simulink library "BibSpielo"  (R2025b)
settings: Solver=VariableStepAuto  StartTime=0.0  StopTime=10.0  RelTol=1e-3
settings Model: Creator=henni  LastModifiedBy=henni

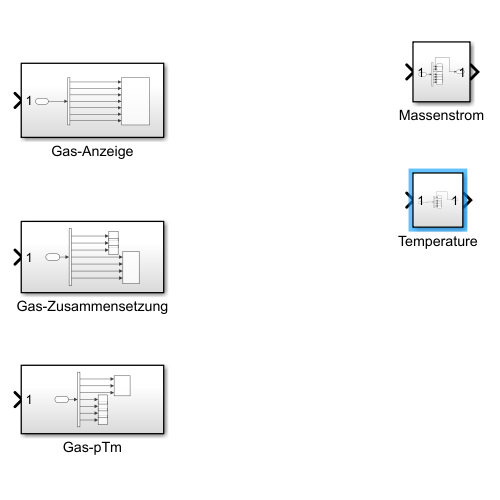
[thumbnail: Simulink's stored preview of the top-level diagram]
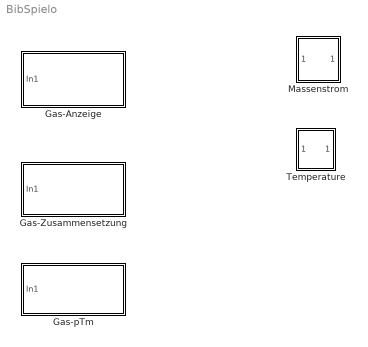
== system BibSpielo ==
  Gas-Anzeige : Subsystem
  Gas-Zusammensetzung : Subsystem
  Gas-pTm : Subsystem
  Massenstrom : Subsystem
  Temperature : Subsystem

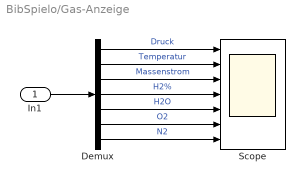
== system BibSpielo/Gas-Anzeige ==
  In1 : Inport
  Demux : Demux  Outputs=7
  Scope : Scope  NumInputPorts=7
  wires:
  Demux/3 -> Scope/3  "Massenstrom"
  Demux/2 -> Scope/2  "Temperatur"
  Demux/1 -> Scope/1  "Druck"
  Demux/7 -> Scope/7  "N2"
  Demux/4 -> Scope/4  "H2%"
  Demux/6 -> Scope/6  "O2"
  Demux/5 -> Scope/5  "H2O"
  In1/1 -> Demux/1

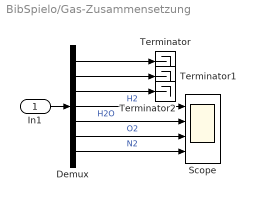
== system BibSpielo/Gas-Zusammensetzung ==
  In1 : Inport
  Demux : Demux  Outputs=7
  Scope : Scope  NumInputPorts=4
  Terminator : Terminator
  Terminator1 : Terminator
  Terminator2 : Terminator
  wires:
  Demux/6 -> Scope/3  "O2"
  Demux/7 -> Scope/4  "N2"
  In1/1 -> Demux/1
  Demux/2 -> Terminator1/1
  Demux/1 -> Terminator/1
  Demux/4 -> Scope/1  "H2"
  Demux/3 -> Terminator2/1
  Demux/5 -> Scope/2  "H2O"

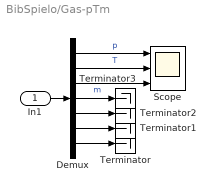
== system BibSpielo/Gas-pTm ==
  In1 : Inport
  Demux : Demux  Outputs=7
  Scope : Scope  NumInputPorts=3
      settings: DataLoggingVariableName=ScopeData2
  Terminator{,1..3} (4 alike) : Terminator
  wires:
  Demux/6 -> Terminator1/1
  In1/1 -> Demux/1
  Demux/3 -> Scope/3  "m"
  Demux/1 -> Scope/1  "p"
  Demux/2 -> Scope/2  "T"
  Demux/4 -> Terminator3/1
  Demux/5 -> Terminator2/1
  Demux/7 -> Terminator/1

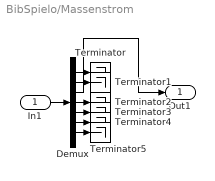
== system BibSpielo/Massenstrom ==
  In1 : Inport
  Demux : Demux  Outputs=7
  Terminator{,1..5} (6 alike) : Terminator
  Out1 : Outport
  wires:
  Demux/2 -> Terminator1/1
  In1/1 -> Demux/1
  Demux/4 -> Terminator2/1
  Demux/6 -> Terminator4/1
  Demux/5 -> Terminator3/1
  Demux/1 -> Terminator/1
  Demux/7 -> Terminator5/1
  Demux/3 -> Out1/1

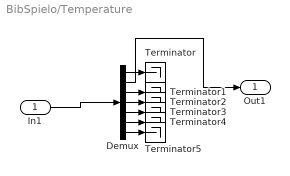
== system BibSpielo/Temperature ==
  In1 : Inport
  Demux : Demux  Outputs=7
  Terminator{,1..5} (6 alike) : Terminator
  Out1 : Outport
  wires:
  Demux/1 -> Terminator/1
  Demux/7 -> Terminator5/1
  Demux/6 -> Terminator4/1
  In1/1 -> Demux/1
  Demux/5 -> Terminator3/1
  Demux/4 -> Terminator2/1
  Demux/3 -> Terminator1/1
  Demux/2 -> Out1/1
